simulink model "simulinkTutorial2"  (Simulink 7.7)
settings: Solver=ode45  StartTime=0.0  StopTime=30  RelTol=1e-3
settings Model: Creator=jiannianweng  LastModifiedBy=jiannianweng

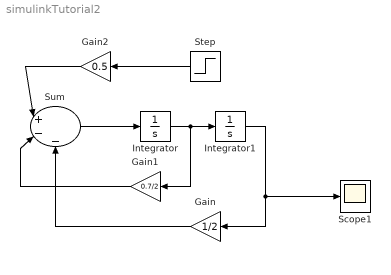
== system simulinkTutorial2 ==
  Gain : Gain  Gain=1/2
  Gain1 : Gain  Gain=0.7/2
  Gain2 : Gain  Gain=0.5
  Integrator : Integrator
  Integrator1 : Integrator
  Scope1 : Scope
  Step : Step  SampleTime=0
  Sum : Sum  Inputs=|+--
  wires:
  Integrator/1 -> Integrator1/1, Gain1/1
  Sum/1 -> Integrator/1
  Integrator1/1 -> Gain/1, Scope1/1
  Gain/1 -> Sum/3
  Gain1/1 -> Sum/2
  Gain2/1 -> Sum/1
  Step/1 -> Gain2/1
